simulink model "BT2"  (R2019a)
settings: Solver=ode5  StartTime=0.0  StopTime=20  FixedStep=0.001  RelTol=1e-3
libraries: fuzblock x1
settings Model: Creator=ASUS  LastModifiedBy=ASUS

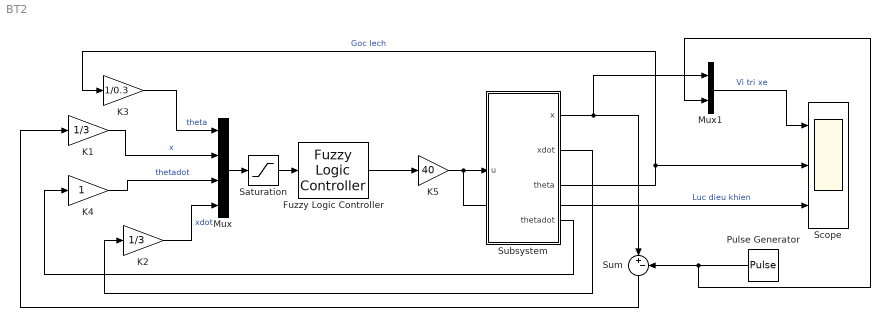
== system BT2 ==
  Fuzzy Logic Controller : fuzblock/Fuzzy Logic  Controller  FIS='bt2.fis'  OutputSampleNumber=101  DataType=double  FuzzifiedInputs=off  RuleFiringStrengths=off  RuleOutputs=off  AggregatedOutputs=off  SimulateUsing=Interpreted execution  OutOfRangeInputValueMessage=warning  NoRuleFiredMessage=warning  EmptyOutputFuzzySetMessage=warning
  K1 : Gain  Gain=1/3
  K2 : Gain  Gain=1/3
  K3 : Gain  Gain=1/0.3
  K4 : Gain
  K5 : Gain  Gain=40
  Mux : Mux
  Mux1 : Mux  Inputs=2
  Pulse Generator : DiscretePulseGenerator  PulseType=Time based  Period=20  PulseWidth=50
  Saturation : Saturate  UpperLimit=1  LowerLimit=-1
  Scope : Scope  NumInputPorts=3
  Subsystem : Subsystem  mask{M=1, m_=0.1, l=0.5, g=9.81, x0=1, xdot0=1.5, theta0=0.2, thetadot0=0.3}
      mask prompts: M "Trong luong xe (kg)"; m_ "Trong luong con lac (kg)"; l "Chieu dai con lac (m)"; g "Gia toc trong truong (m/s2)"; x0 "Vi tri ban dau (m)"; xdot0 "Van toc ban dau (m/s)"; theta0 "Goc ban dau( rad)"; thetadot0 "Van toc goc ban dau (rad/s)"
  Sum : Sum  Inputs=|+-
  wires:
  Saturation/1 -> Fuzzy Logic Controller/1
  K5/1 -> Scope/3, Subsystem/1(u)  "Luc dieu khien"
  Mux/1 -> Saturation/1
  Fuzzy Logic Controller/1 -> K5/1
  Subsystem/1(x) -> Sum/1, Mux1/1
  Subsystem/3(theta) -> K3/1, Scope/2  "Goc lech"
  Subsystem/4(thetadot) -> K4/1
  Subsystem/2(xdot) -> K2/1
  Pulse Generator/1 -> Sum/2, Mux1/2
  K3/1 -> Mux/1  "theta"
  K1/1 -> Mux/2  "x"
  K4/1 -> Mux/3  "thetadot"
  K2/1 -> Mux/4  "xdot"
  Sum/1 -> K1/1
  Mux1/1 -> Scope/1  "Vi tri xe"

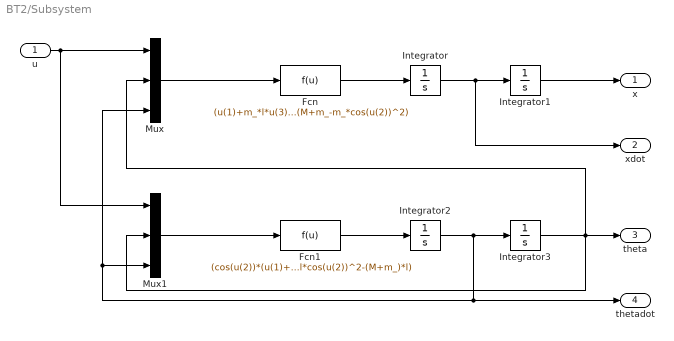
== system BT2/Subsystem ==
  u : Inport
  Fcn : Fcn  Expr=(u(1)+m_*l*u(3)^2*sin(u(2))-m_*g*sin(u(2))*cos(u(2)))/(M+m_-m_*cos(u(2))^2)
  Fcn1 : Fcn  Expr=(cos(u(2))*(u(1)+m_*g*u(3)^2*sin(u(2)))-(M+m_)*(g*sin(u(2))))/(m_*l*cos(u(2))^2-(M+m_)*l)
  Integrator : Integrator  InitialCondition=xdot0
  Integrator1 : Integrator  InitialCondition=x0
  Integrator2 : Integrator  InitialCondition=thetadot0
  Integrator3 : Integrator  InitialCondition=theta0
  Mux : Mux  Inputs=3
  Mux1 : Mux  Inputs=3
  x : Outport
  xdot : Outport  Port=2
  theta : Outport  Port=3
  thetadot : Outport  Port=4
  wires:
  u/1 -> Mux1/1, Mux/1
  Fcn/1 -> Integrator/1
  Integrator/1 -> xdot/1, Integrator1/1
  Integrator1/1 -> x/1
  Mux/1 -> Fcn/1
  Integrator3/1 -> Mux/2, Mux1/2, theta/1
  Integrator2/1 -> Mux/3, Mux1/3, thetadot/1, Integrator3/1
  Fcn1/1 -> Integrator2/1
  Mux1/1 -> Fcn1/1
